simulink library "magnetorquer_lib"  (R2016b)
settings: Solver=VariableStepAuto  StartTime=0.0  StopTime=10.0  RelTol=1e-3
undefined symbols (not defined in the file): sim_params
libraries: simulink x1
settings Model: Creator=Taylor  LastModifiedBy=taylorreynolds

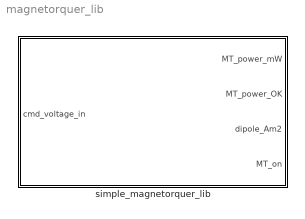
== system magnetorquer_lib ==
  simple_magnetorquer_lib : Subsystem  mask{A=sim_params.actuators.magnetorquer.area_x, N=sim_params.actuators.magnetorquer.num_turns_x, mu=sim_params.actuators.magnetorquer.mu_x, Linv=1/sim_params.actuators.magnetorquer.inductance_x, R=sim_params.actuators.magnetorquer.resistance_x, UpperLimit=sim_params.actuators.magnetorquer.max_dipole, LowerLimit=-sim_params.actuators.magnetorquer.max_dipole}
      mask prompts: A "Simulink:blkprm_prompts:GainGain"; N "Simulink:blkprm_prompts:GainGain"; mu "Simulink:blkprm_prompts:GainGain"; Linv "Simulink:blkprm_prompts:GainGain"; R "Simulink:blkprm_prompts:GainGain"; UpperLimit "Simulink:blkprm_prompts:SaturateUpLim"; LowerLimit "Simulink:blkprm_prompts:SaturateLowLim"
      mask TypeOptions A: A/Gain
      mask TypeOptions N: N/Gain
      mask TypeOptions mu: mu/Gain
      mask TypeOptions Linv: Gain/Gain
      mask TypeOptions R: Gain1/Gain
      mask TypeOptions UpperLimit: Saturation/UpperLimit
      mask TypeOptions LowerLimit: Saturation/LowerLimit
      mask DialogControl Control2 Prompt: Takes commanded voltage and spits out the resulting dipole moment. Computed according to $$ m = \mu N A I $$, where $ \mu  = k_{eff} \mu_{rel} \mu_0$.

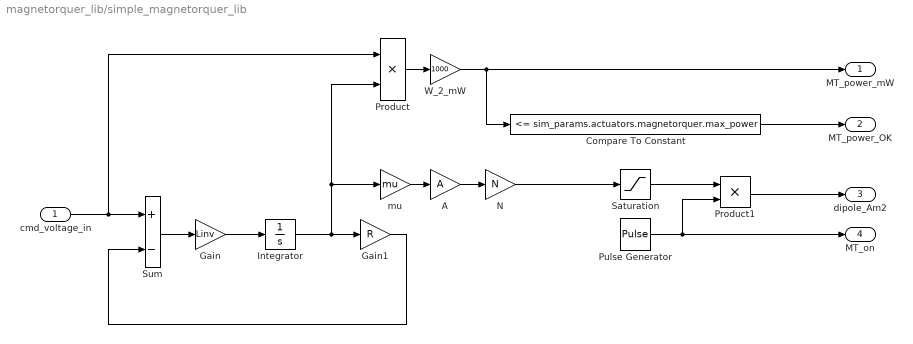
== system magnetorquer_lib/simple_magnetorquer_lib ==
  cmd_voltage_in : Inport
  A : Gain  Gain=A
  Compare To Constant : simulink/Logic and Bit Operations/Compare To Constant  relop=<=  const=sim_params.actuators.magnetorquer.max_power  OutDataTypeStr=boolean
  Gain : Gain  Gain=Linv
  Gain1 : Gain  Gain=R
  Integrator : Integrator  InitialCondition=sim_params.actuators.magnetorquer.ic.current
  N : Gain  Gain=N
  Product : Product
  Product1 : Product
  Pulse Generator : DiscretePulseGenerator  PulseType=Time based  Period=1  PulseWidth=fsw_params.actuators.magnetorquer.actuation_time_pct
  Saturation : Saturate  UpperLimit=UpperLimit  LowerLimit=LowerLimit
  Sum : Sum  Inputs=+-
  W_2_mW : Gain  Gain=1000
  mu : Gain  Gain=mu
  MT_power_mW : Outport
  MT_power_OK : Outport  Port=2
  dipole_Am2 : Outport  Port=3
  MT_on : Outport  Port=4
  wires:
  W_2_mW/1 -> MT_power_mW/1, Compare To Constant/1
  Compare To Constant/1 -> MT_power_OK/1
  Gain1/1 -> Sum/2
  Sum/1 -> Gain/1
  Integrator/1 -> Gain1/1, mu/1, Product/2
  Product/1 -> W_2_mW/1
  Gain/1 -> Integrator/1
  cmd_voltage_in/1 -> Product/1, Sum/1
  N/1 -> Saturation/1
  Pulse Generator/1 -> MT_on/1, Product1/2
  A/1 -> N/1
  mu/1 -> A/1
  Saturation/1 -> Product1/1
  Product1/1 -> dipole_Am2/1
